simulink model "my_quadrotor_adrc_nolimit"  (R2017b)
settings: Solver=FixedStepAuto  StartTime=0.0  StopTime=100  FixedStep=0.002  RelTol=1e-3
settings Model: Creator=apple  LastModifiedBy=apple
settings DebuggingCC: AlgebraicLoopMsg=none

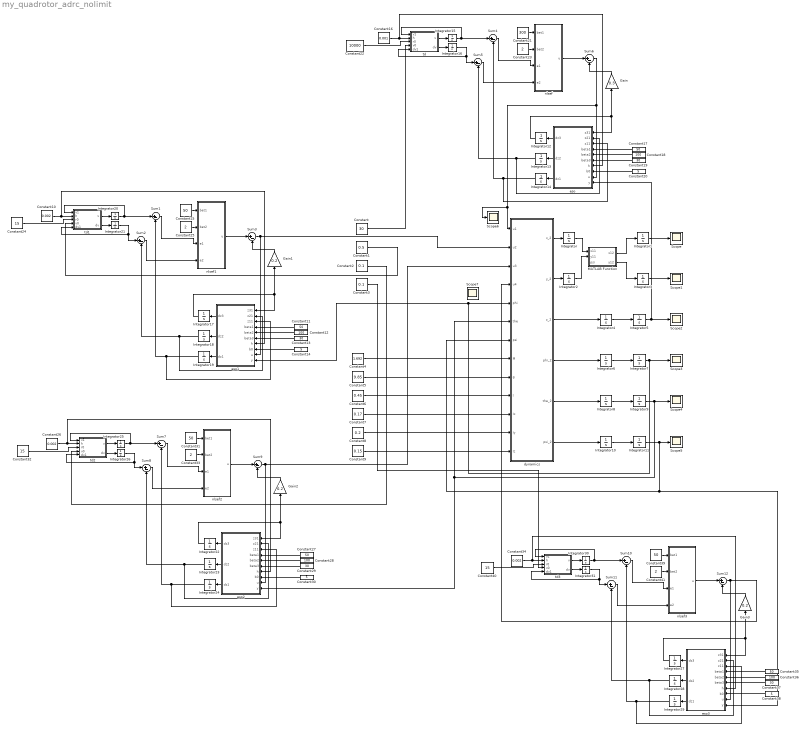
== system my_quadrotor_adrc_nolimit ==
  Constant{,13,19,29,37} (5 alike) : Constant  Value=30
  Constant1 : Constant  Value=0.5
  Constant10 : Constant  Value=0.002
  Constant{11,15,17,27,31,35,39} (7 alike) : Constant  Value=50
  Constant{12,18,28,36} (4 alike) : Constant  Value=100
  Constant{14,20,30,38} (4 alike) : Constant  Value=5
  Constant16 : Constant  Value=0.001
  Constant2 : Constant  Value=0.1
  Constant21 : Constant  Value=300
  Constant22 : Constant  Value=10000
  Constant{23,25,33,41} (4 alike) : Constant  Value=2
  Constant24 : Constant  Value=15
  Constant26 : Constant  Value=0.002
  Constant3 : Constant  Value=0.1
  Constant32 : Constant  Value=15
  Constant34 : Constant  Value=0.002
  Constant4 : Constant  Value=1.692
  Constant40 : Constant  Value=15
  Constant5 : Constant  Value=9.85
  Constant6 : Constant  Value=0.45
  Constant7 : Constant  Value=0.17
  Constant8 : Constant  Value=0.2
  Constant9 : Constant  Value=0.15
  Gain : Gain  Gain=0.3
  Gain1 : Gain  Gain=0.2
  Gain2 : Gain  Gain=0.2
  Gain3 : Gain  Gain=0.2
  Integrator{,1..31} (32 alike) : Integrator
  MATLAB Function : MATLAB Function  TreatAsAtomicUnit=on
  Scope{,1..7} (8 alike) : Scope
  Sum{1..12} (12 alike) : Sum  Inputs=|+-
  dynamics : MATLAB Function  TreatAsAtomicUnit=on
  eso : MATLAB Function  TreatAsAtomicUnit=on
  eso1 : MATLAB Function  TreatAsAtomicUnit=on
  eso2 : MATLAB Function  TreatAsAtomicUnit=on
  eso3 : MATLAB Function  TreatAsAtomicUnit=on
  nlsef : MATLAB Function  TreatAsAtomicUnit=on
  nlsef1 : MATLAB Function  TreatAsAtomicUnit=on
  nlsef2 : MATLAB Function  TreatAsAtomicUnit=on
  nlsef3 : MATLAB Function  TreatAsAtomicUnit=on
  td : MATLAB Function  TreatAsAtomicUnit=on
  td1 : MATLAB Function  TreatAsAtomicUnit=on
  td2 : MATLAB Function  TreatAsAtomicUnit=on
  td3 : MATLAB Function  TreatAsAtomicUnit=on
  wires:
  Integrator4/1 -> Integrator5/1
  Integrator5/1 -> Scope2/1, eso/10(y)
  dynamics/3(z_2) -> Integrator4/1
  Integrator6/1 -> Integrator7/1
  Integrator7/1 -> Scope3/1, eso1/10(y), dynamics/5(phi)
  dynamics/4(phi_2) -> Integrator6/1
  Integrator8/1 -> Integrator9/1
  Integrator9/1 -> eso2/10(y), dynamics/6(the), Scope4/1
  dynamics/5(the_2) -> Integrator8/1
  Integrator10/1 -> Integrator11/1
  Integrator11/1 -> eso3/10(y), dynamics/7(psi), Scope5/1
  dynamics/6(psi_2) -> Integrator10/1
  Constant4/1 -> dynamics/8(M)
  Constant5/1 -> dynamics/9(g)
  Constant6/1 -> dynamics/10(l)
  Constant7/1 -> dynamics/11(Ix)
  Constant8/1 -> dynamics/12(Iy)
  Constant9/1 -> dynamics/13(Iz)
  nlsef/1(u) -> Sum6/1
  Constant17/1 -> eso/4(beta1)
  Constant19/1 -> eso/6(beta3)
  Constant18/1 -> eso/5(beta2)
  Constant23/1 -> nlsef/2(bet2)
  eso/2(dz2) -> Integrator13/1
  Constant22/1 -> td/3(r0)
  eso/3(dz1) -> Integrator14/1
  Integrator13/1 -> Sum5/2, eso/2(z21)
  eso/1(dz3) -> Integrator12/1
  Integrator14/1 -> Sum4/2, eso/3(z11)
  Constant20/1 -> eso/8(b0)
  Sum5/1 -> nlsef/4(e2)
  Sum4/1 -> nlsef/3(e1)
  Constant21/1 -> nlsef/1(bet1)
  Integrator16/1 -> Sum5/1, td/5(dv1)
  td/2(dv) -> Integrator16/1
  Integrator15/1 -> Sum4/1, td/1(v1)
  Integrator12/1 -> eso/1(z31), Gain/1
  Constant16/1 -> eso/7(h), td/2(h)
  td/1(v) -> Integrator15/1
  Gain/1 -> Sum6/2
  Constant/1 -> td/4(v0)
  Integrator17/1 -> eso1/1(z31), Gain1/1
  eso1/2(dz2) -> Integrator18/1
  Sum3/1 -> dynamics/2(u2), eso1/9(u)
  eso1/1(dz3) -> Integrator17/1
  Constant25/1 -> nlsef1/2(bet2)
  Integrator21/1 -> Sum2/1, td1/5(dv1)
  Integrator20/1 -> Sum1/1, td1/1(v1)
  td1/2(dv) -> Integrator21/1
  Constant11/1 -> eso1/4(beta1)
  eso1/3(dz1) -> Integrator19/1
  Integrator18/1 -> Sum2/2, eso1/2(z21)
  Constant12/1 -> eso1/5(beta2)
  Sum2/1 -> nlsef1/4(e2)
  Constant24/1 -> td1/3(r0)
  Constant13/1 -> eso1/6(beta3)
  td1/1(v) -> Integrator20/1
  Gain1/1 -> Sum3/2
  Constant10/1 -> eso1/7(h), td1/2(h)
  Constant14/1 -> eso1/8(b0)
  Sum1/1 -> nlsef1/3(e1)
  Constant15/1 -> nlsef1/1(bet1)
  nlsef1/1(u) -> Sum3/1
  Integrator19/1 -> Sum1/2, eso1/3(z11)
  Constant1/1 -> td1/4(v0)
  Integrator22/1 -> eso2/1(z31), Gain2/1
  eso2/2(dz2) -> Integrator23/1
  Sum9/1 -> dynamics/3(u3), eso2/9(u)
  eso2/1(dz3) -> Integrator22/1
  Constant33/1 -> nlsef2/2(bet2)
  Integrator26/1 -> Sum8/1, td2/5(dv1)
  Integrator25/1 -> Sum7/1, td2/1(v1)
  td2/2(dv) -> Integrator26/1
  Constant27/1 -> eso2/4(beta1)
  eso2/3(dz1) -> Integrator24/1
  Integrator23/1 -> Sum8/2, eso2/2(z21)
  Constant28/1 -> eso2/5(beta2)
  Sum8/1 -> nlsef2/4(e2)
  Constant32/1 -> td2/3(r0)
  Constant29/1 -> eso2/6(beta3)
  td2/1(v) -> Integrator25/1
  Gain2/1 -> Sum9/2
  Constant26/1 -> eso2/7(h), td2/2(h)
  Constant30/1 -> eso2/8(b0)
  Sum7/1 -> nlsef2/3(e1)
  Constant31/1 -> nlsef2/1(bet1)
  nlsef2/1(u) -> Sum9/1
  Integrator24/1 -> Sum7/2, eso2/3(z11)
  Constant2/1 -> td2/4(v0)
  Integrator27/1 -> eso3/1(z31), Gain3/1
  eso3/2(dz2) -> Integrator28/1
  Sum12/1 -> eso3/9(u), dynamics/4(u4)
  eso3/1(dz3) -> Integrator27/1
  Constant41/1 -> nlsef3/2(bet2)
  Integrator31/1 -> Sum11/1, td3/5(dv1)
  Integrator30/1 -> Sum10/1, td3/1(v1)
  td3/2(dv) -> Integrator31/1
  Constant35/1 -> eso3/4(beta1)
  eso3/3(dz1) -> Integrator29/1
  Integrator28/1 -> Sum11/2, eso3/2(z21)
  Constant36/1 -> eso3/5(beta2)
  Sum11/1 -> nlsef3/4(e2)
  Constant40/1 -> td3/3(r0)
  Constant37/1 -> eso3/6(beta3)
  td3/1(v) -> Integrator30/1
  Gain3/1 -> Sum12/2
  Constant34/1 -> eso3/7(h), td3/2(h)
  Constant38/1 -> eso3/8(b0)
  Sum10/1 -> nlsef3/3(e1)
  Constant39/1 -> nlsef3/1(bet1)
  nlsef3/1(u) -> Sum12/1
  Integrator29/1 -> Sum10/2, eso3/3(z11)
  Constant3/1 -> td3/4(v0)
  Integrator2/1 -> MATLAB Function/2(y11)
  dynamics/2(y_2) -> Integrator2/1
  dynamics/1(x_2) -> Integrator/1
  Integrator/1 -> MATLAB Function/1(x11)
  MATLAB Function/1(x12) -> Integrator1/1
  MATLAB Function/2(y12) -> Integrator3/1
  Integrator1/1 -> Scope/1
  Integrator3/1 -> Scope1/1
  Sum6/1 -> Scope6/1, dynamics/1(u1), eso/9(u)

== matlab function my_quadrotor_adrc_nolimit/td ==
  data: v1 input; h input; r0 input; v0 input; dv1 input; v output; dv output
function [v,dv] = td(v1,h,r0,v0,dv1)

%fh = fhan(v1 - v0,dv1,r0,h)
d = r0 * h * h;
a0 = h * dv1;
y = v1 - v0 + a0;
a1 = sqrt(d * (d + 8 * abs(y)));
a2 = a0 + sign(y) * (a1 - d)/2;
a = (a0 + y -a2) * (sign(y + d) - sign(y - d))/2 + a2;
fh = -r0 * (a/d - sign(a)) * (sign(a + d) - sign(a - d))/2 - r0 * sign(a);

v = dv1;
dv = fh;
%v = v1 + h * dv1;
%dv = dv1 + h * fh;
end

== matlab function my_quadrotor_adrc_nolimit/dynamics ==
  data: u1 input; x_2 output; u2 input; u3 input; u4 input; phi input; the input; psi input; M input; g input; l input; Ix input; Iy input; Iz input; y_2 output; z_2 output; phi_2 output; the_2 output; psi_2 output
function [x_2, y_2, z_2, phi_2, the_2, psi_2] = dynamics(u1,u2,u3,u4,phi,the,psi,M,g,l,Ix,Iy,Iz)
x_2 = u1*(cos(phi)*sin(the)*cos(psi)+sin(phi)*sin(psi))/M;
y_2 = u1*(cos(phi)*sin(the)*cos(psi)-sin(phi)*sin(psi))/M;
z_2 = -g+u1*(cos(the)*cos(phi))/M;
phi_2 = l*u2/Ix;
the_2 = l*u3/Iy;
psi_2 = l*u4/Iz;

== matlab function my_quadrotor_adrc_nolimit/eso1 ==
  data: dz3 output; dz2 output; z31 input; z21 input; z11 input; beta1 input; beta2 input; beta3 input; h input; b0 input; dz1 output; u input; y input
function [dz3,dz2,dz1] = eso(z31,z21,z11,beta1,beta2,beta3,h,b0,u,y)

%ts = 0.001;
e = z11 - y;
dz1 = z21 - beta1 * e;
dz2 = z31 - beta2 * fal(e,0.5,h) + b0 * u;
dz3 = -beta3 * fal(e,0.25,h);

end

function fe = fal(error,pow,threshold)
if abs(error) > threshold
    fe = (abs(error))^pow * sign(error);
else
    fe = error * threshold^(pow - 1);
end
end

== matlab function my_quadrotor_adrc_nolimit/nlsef1 ==
  data: bet1 input; bet2 input; e1 input; u output; e2 input
function u = nlsef(bet1,bet2,e1,e2)

a1 = 0.5;
a2 = 0.75;
delta1 = 0.001;
delta2 = 0.005;
u = bet1 * fal(e1,a1,delta1) + bet2 * fal(e2,a2,delta2);
end

function fe = fal(error,pow,threshold)
if abs(error) > threshold
    fe = (abs(error))^pow * sign(error);
else
    fe = error * threshold^(pow - 1);
end
end

== matlab function my_quadrotor_adrc_nolimit/td1 ==
  data: v1 input; h input; r0 input; v0 input; dv1 input; v output; dv output
function [v,dv] = td(v1,h,r0,v0,dv1)

%fh = fhan(v1 - v0,dv1,r0,h)
d = r0 * h * h;
a0 = h * dv1;
y = v1 - v0 + a0;
a1 = sqrt(d * (d + 8 * abs(y)));
a2 = a0 + sign(y) * (a1 - d)/2;
a = (a0 + y -a2) * (sign(y + d) - sign(y - d))/2 + a2;
fh = -r0 * (a/d - sign(a)) * (sign(a + d) - sign(a - d))/2 - r0 * sign(a);

v = dv1;
dv = fh;
%v = v1 + h * dv1;
%dv = dv1 + h * fh;
end

== matlab function my_quadrotor_adrc_nolimit/nlsef ==
  data: bet1 input; bet2 input; e1 input; u output; e2 input
function u = nlsef(bet1,bet2,e1,e2)

a1 = 0.5;
a2 = 0.75;
delta1 = 0.001;
delta2 = 0.001;
u = bet1 * fal(e1,a1,delta1) + bet2 * fal(e2,a2,delta2);
end

function fe = fal(error,pow,threshold)
if abs(error) > threshold
    fe = (abs(error))^pow * sign(error);
else
    fe = error * threshold^(pow - 1);
end
end

== matlab function my_quadrotor_adrc_nolimit/eso2 ==
  data: dz3 output; dz2 output; z31 input; z21 input; z11 input; beta1 input; beta2 input; beta3 input; h input; b0 input; dz1 output; u input; y input
function [dz3,dz2,dz1] = eso(z31,z21,z11,beta1,beta2,beta3,h,b0,u,y)

%ts = 0.001;
e = z11 - y;
dz1 = z21 - beta1 * e;
dz2 = z31 - beta2 * fal(e,0.5,h) + b0 * u;
dz3 = -beta3 * fal(e,0.25,h);

end

function fe = fal(error,pow,threshold)
if abs(error) > threshold
    fe = (abs(error))^pow * sign(error);
else
    fe = error * threshold^(pow - 1);
end
end

== matlab function my_quadrotor_adrc_nolimit/nlsef2 ==
  data: bet1 input; bet2 input; e1 input; u output; e2 input
function u = nlsef(bet1,bet2,e1,e2)

a1 = 0.5;
a2 = 0.75;
delta1 = 0.001;
delta2 = 0.005;
u = bet1 * fal(e1,a1,delta1) + bet2 * fal(e2,a2,delta2);
end

function fe = fal(error,pow,threshold)
if abs(error) > threshold
    fe = (abs(error))^pow * sign(error);
else
    fe = error * threshold^(pow - 1);
end
end

== matlab function my_quadrotor_adrc_nolimit/eso ==
  data: dz3 output; dz2 output; z31 input; z21 input; z11 input; beta1 input; beta2 input; beta3 input; h input; b0 input; dz1 output; u input; y input
function [dz3,dz2,dz1] = eso(z31,z21,z11,beta1,beta2,beta3,h,b0,u,y)

%ts = 0.001;
e = z11 - y;
dz1 = z21 - beta1 * e;
dz2 = z31 - beta2 * fal(e,0.5,h) + b0 * u;
dz3 = -beta3 * fal(e,0.25,h);

end

function fe = fal(error,pow,threshold)
if abs(error) > threshold
    fe = (abs(error))^pow * sign(error);
else
    fe = error * threshold^(pow - 1);
end
end

== matlab function my_quadrotor_adrc_nolimit/td2 ==
  data: v1 input; h input; r0 input; v0 input; dv1 input; v output; dv output
function [v,dv] = td(v1,h,r0,v0,dv1)

%fh = fhan(v1 - v0,dv1,r0,h)
d = r0 * h * h;
a0 = h * dv1;
y = v1 - v0 + a0;
a1 = sqrt(d * (d + 8 * abs(y)));
a2 = a0 + sign(y) * (a1 - d)/2;
a = (a0 + y -a2) * (sign(y + d) - sign(y - d))/2 + a2;
fh = -r0 * (a/d - sign(a)) * (sign(a + d) - sign(a - d))/2 - r0 * sign(a);

v = dv1;
dv = fh;
%v = v1 + h * dv1;
%dv = dv1 + h * fh;
end

== matlab function my_quadrotor_adrc_nolimit/eso3 ==
  data: dz3 output; dz2 output; z31 input; z21 input; z11 input; beta1 input; beta2 input; beta3 input; h input; b0 input; dz1 output; u input; y input
function [dz3,dz2,dz1] = eso(z31,z21,z11,beta1,beta2,beta3,h,b0,u,y)

%ts = 0.001;
e = z11 - y;
dz1 = z21 - beta1 * e;
dz2 = z31 - beta2 * fal(e,0.5,h) + b0 * u;
dz3 = -beta3 * fal(e,0.25,h);

end

function fe = fal(error,pow,threshold)
if abs(error) > threshold
    fe = (abs(error))^pow * sign(error);
else
    fe = error * threshold^(pow - 1);
end
end

== matlab function my_quadrotor_adrc_nolimit/nlsef3 ==
  data: bet1 input; bet2 input; e1 input; u output; e2 input
function u = nlsef(bet1,bet2,e1,e2)

a1 = 0.5;
a2 = 0.75;
delta1 = 0.001;
delta2 = 0.005;
u = bet1 * fal(e1,a1,delta1) + bet2 * fal(e2,a2,delta2);
end

function fe = fal(error,pow,threshold)
if abs(error) > threshold
    fe = (abs(error))^pow * sign(error);
else
    fe = error * threshold^(pow - 1);
end
end

== matlab function my_quadrotor_adrc_nolimit/td3 ==
  data: v1 input; h input; r0 input; v0 input; dv1 input; v output; dv output
function [v,dv] = td(v1,h,r0,v0,dv1)

%fh = fhan(v1 - v0,dv1,r0,h)
d = r0 * h * h;
a0 = h * dv1;
y = v1 - v0 + a0;
a1 = sqrt(d * (d + 8 * abs(y)));
a2 = a0 + sign(y) * (a1 - d)/2;
a = (a0 + y -a2) * (sign(y + d) - sign(y - d))/2 + a2;
fh = -r0 * (a/d - sign(a)) * (sign(a + d) - sign(a - d))/2 - r0 * sign(a);

v = dv1;
dv = fh;
%v = v1 + h * dv1;
%dv = dv1 + h * fh;
end

== matlab function my_quadrotor_adrc_nolimit/MATLAB Function ==
  data: x11 input; x12 output; y11 input; psi input; y12 output
function [x12,y12] = rot(x11,y11,psi)

x12 = x11 * cos(psi) - y11 * sin(psi);
y12 = x11 * sin(psi) + y11 * cos(psi);
